simulink model "LEGO_SW_simp"  (R2023a)
settings: Solver=FixedStepAuto  StartTime=0.0  StopTime=45  FixedStep=1e-3  RelTol=1e-3  EnableMultiTasking=on
values from neighbouring files (symbols this model uses):
  A1 = [0,0,1,0 ... (first row only)    [run_LEGO_SW.m]
  A2 = [0,1;0,-W^2/(2*R^2)*(Kfrac+b+b_bar)/Denom]    [run_LEGO_SW.m]
  B1 = [0;0;2*(M*R*L+M*L^2+Jpsi)*Kt/Rdc/q;-2*((2*m+M)*R^2+2*J+M*R*L)*Kt/Rdc/q]    [run_LEGO_SW.m]
  B2 = [0;-W/R*Kt/Rdc/Denom]    [run_LEGO_SW.m]
  C1 = [1,0,0,0;0,0,0,1]    [run_LEGO_SW.m]
  C2 = [1,0]    [run_LEGO_SW.m]
  D1 = [0;0]    [run_LEGO_SW.m]
  D2 = 0    [run_LEGO_SW.m]
  KPphi = 6    [run_LEGO_SW.m]
undefined symbols (not defined in the file or in its folder): Kpp, sigbuilder_block
settings Model: Creator=KostasM  LastModifiedBy=lab5
settings SolverCC: AlgebraicLoopSolver=TrustRegion
settings DataIOCC: LimitDataPoints=on  ReturnWorkspaceOutputs=off
settings OptimizationCC: LifeSpan=inf
settings DebuggingCC: UnconnectedInputMsg=warning  UnconnectedOutputMsg=warning  UnconnectedLineMsg=warning  AllowSymbolicDim=off  SFUnexpectedBacktrackingDiag=warning  SFNoUnconditionalDefaultTransitionDiag=warning  SFExecutionAtInitializationDiag=none  ArithmeticOperatorsInVariantConditions=warning
settings ModelReferenceCC: EnableRefExpFcnMdlSchedulingChecks=on  PropagateSignalLabelsOutOfModel=off
settings SFSimCC: SimUseLocalCustomCode=off  CustomCodeUndefinedFunction=UseInterfaceOnly
settings RTWCC: RTWUseLocalCustomCode=off  DLArmComputeVersion=19.05
settings CodeAppCC: StateflowObjectComments=on
settings GRTTargetCC: TargetLangStandard=C89/C90 (ANSI)
settings ConfigComp: CovMetricSettings=dw  CovSaveCumulativeToWorkspaceVar=on  CovSaveSingleToWorkspaceVar=on  CovExternalEMLEnable=off

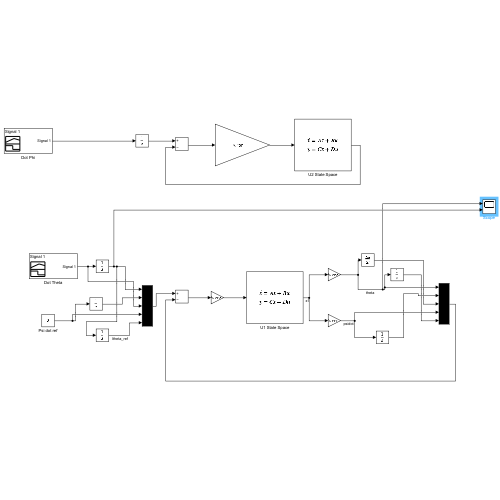
[thumbnail: Simulink's stored preview of the top-level diagram]
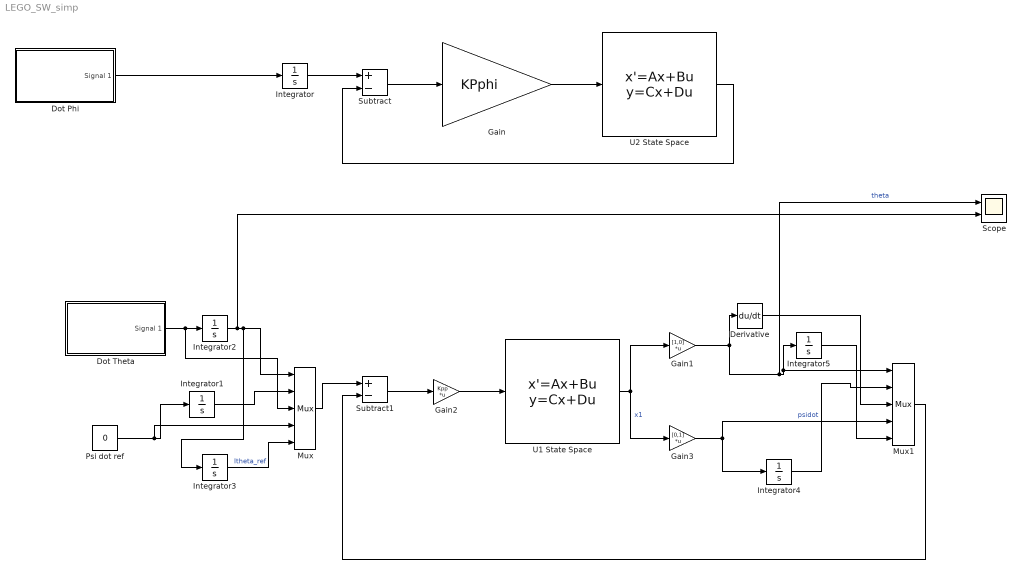
== system LEGO_SW_simp ==
  Derivative : Derivative
  Dot Phi : Subsystem  Tag=STV Subsys  LoadFcn=sigbuilder_block('load');  StartFcn=sigbuilder_block('start');  StopFcn=sigbuilder_block('stop');  ClipboardFcn=sigbuilder_block('clipboard');  mask(Sigbuilder block){tuvar=[0:10]}
      mask help: Sigbuilder GUI
      mask init:
      | if ~strcmp(get_param(bdroot(gcbh),'SimulationStatus'),'stopped') tuvar = sigbuilder_block('maskInit'); end
      settings: CopyFcn=sigbuilder_block('copy');  DeleteFcn=sigbuilder_block('delete');  ModelCloseFcn=sigbuilder_block('modelClose');  PreSaveFcn=sigbuilder_block('preSave');  PauseFcn=sigbuilder_block('pause')  ContinueFcn=sigbuilder_block('continue')  NameChangeFcn=sigbuilder_block('namechange');  OpenFcn=sigbuilder_block('open',[181.5 38.5 516 349.5 ]);  CloseFcn=sigbuilder_block('close');
      mask Display: plot(0, 0, 100, 100,[2, 2, 32, 32, 2], [68, 8, 8, 68, 68],[32, 2], [38, 38], [32, 19, 2],[53, 60, 44], [32, 17, 17, 2],[16, 16, 31, 31]);txt = getActiveGroup(gcbh);text(2, 100, txt,'verticalAlignment', 'top');
  Dot Theta : Subsystem  Tag=STV Subsys  LoadFcn=sigbuilder_block('load',[181.5 38.5 516 349.5 ]);  StartFcn=sigbuilder_block('start');  StopFcn=sigbuilder_block('stop');  ClipboardFcn=sigbuilder_block('clipboard');  mask(Sigbuilder block){tuvar=[0:10]}
      mask help: Sigbuilder GUI
      mask init:
      | if ~strcmp(get_param(bdroot(gcbh),'SimulationStatus'),'stopped') tuvar = sigbuilder_block('maskInit'); end
      settings: CopyFcn=sigbuilder_block('copy');  DeleteFcn=sigbuilder_block('delete');  ModelCloseFcn=sigbuilder_block('modelClose');  PreSaveFcn=sigbuilder_block('preSave');  PauseFcn=sigbuilder_block('pause')  ContinueFcn=sigbuilder_block('continue')  NameChangeFcn=sigbuilder_block('namechange');  OpenFcn=sigbuilder_block('open',[181.5 38.5 516 349.5 ]);  CloseFcn=sigbuilder_block('close');
      mask Display: plot(0, 0, 100, 100,[2, 2, 32, 32, 2], [68, 8, 8, 68, 68],[32, 2], [38, 38], [32, 19, 2],[53, 60, 44], [32, 17, 17, 2],[16, 16, 31, 31]);txt = getActiveGroup(gcbh);text(2, 100, txt,'verticalAlignment', 'top');
  Gain : Gain  Gain=KPphi
  Gain1 : Gain  Gain=[1,0]  Multiplication=Matrix(K*u) (u vector)
  Gain2 : Gain  Gain=Kpp  Multiplication=Matrix(K*u) (u vector)
  Gain3 : Gain  Gain=[0,1]  Multiplication=Matrix(K*u) (u vector)
  Integrator{,1..5} (6 alike) : Integrator
  Mux : Mux  Inputs=5
  Mux1 : Mux  Inputs=5
  Psi dot ref : Constant  Value=0
  Scope : Scope  NumInputPorts=2
  Subtract : Sum  Inputs=+-
  Subtract1 : Sum  Inputs=+-
  U1 State Space : StateSpace  A=A1  B=B1  C=C1  D=D1  InitialCondition=0
  U2 State Space : StateSpace  A=A2  B=B2  C=C2  D=D2  InitialCondition=0
  wires:
  Dot Phi/1(Signal 1) -> Integrator/1
  Dot Theta/1(Signal 1) -> Mux/3, Integrator2/1
  Integrator/1 -> Subtract/1
  Subtract/1 -> Gain/1
  Gain/1 -> U2 State Space/1
  U2 State Space/1 -> Subtract/2
  Psi dot ref/1 -> Mux/4, Integrator1/1
  Integrator2/1 -> Scope/2, Integrator3/1, Mux/1
  Mux/1 -> Subtract1/1
  Subtract1/1 -> Gain2/1
  Integrator1/1 -> Mux/2
  Integrator3/1 -> Mux/5  "Itheta_ref"
  Gain1/1 -> Derivative/1, Scope/1, Mux1/1, Integrator5/1  "theta"
  Gain3/1 -> Mux1/4, Integrator4/1  "psidot"
  Integrator4/1 -> Mux1/2
  Derivative/1 -> Mux1/3
  Integrator5/1 -> Mux1/5
  Mux1/1 -> Subtract1/2
  Gain2/1 -> U1 State Space/1
  U1 State Space/1 -> Gain1/1, Gain3/1  "x1"

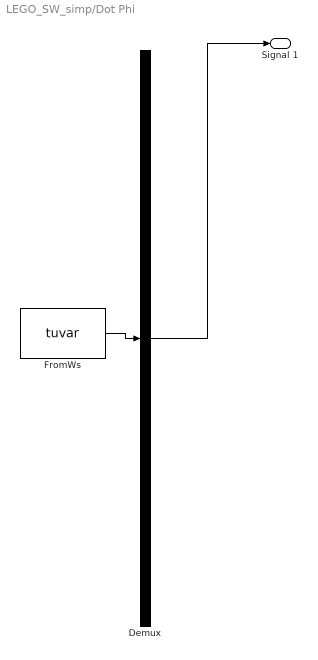
== system LEGO_SW_simp/Dot Phi ==
  Demux : Demux  Tag=STV Demux  Outputs=1
      settings: DisplayOption=none
  FromWs : FromWorkspace  Tag=STV FromWs  VariableName=tuvar
      SigBuilderData=|
      | common.afterFinalStr = 'Extrapolate'
      | common.sampleTime = 0
      | dataSet.timeRange = [0 25]
      | dataSet.name = 'Signal 1'
      | sbobj.Groups.Name = 'Signal 1'
      | sbobj.Groups.Signals.Name = 'Signal 1'
      | sbobj.Groups.Signals.XData = [0 12.5 12.5 25]
      | sbobj.Groups.Signals.YData = [0 0 1 1]
      | sbobj.Groups.TimeRange = [0 25]
  Signal 1 : Outport  Tag=STV Outport
  wires:
  FromWs/1 -> Demux/1
  Demux/1 -> Signal 1/1

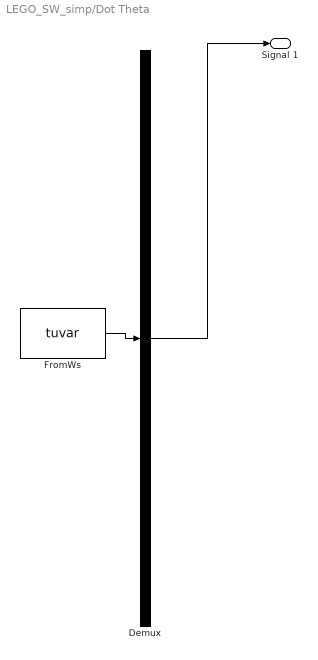
== system LEGO_SW_simp/Dot Theta ==
  Demux : Demux  Tag=STV Demux  Outputs=1
      settings: DisplayOption=none
  FromWs : FromWorkspace  Tag=STV FromWs  VariableName=tuvar
      SigBuilderData=|
      | common.afterFinalStr = 'Extrapolate'
      | common.sampleTime = 0
      | dataSet.timeRange = [0 25]
      | dataSet.name = 'Signal 1'
      | sbobj.Groups.Name = 'Signal 1'
      | sbobj.Groups.Signals.Name = 'Signal 1'
      | sbobj.Groups.Signals.XData = [0 12.5 12.5 25]
      | sbobj.Groups.Signals.YData = [0 0 1 1]
      | sbobj.Groups.TimeRange = [0 25]
  Signal 1 : Outport  Tag=STV Outport
  wires:
  FromWs/1 -> Demux/1
  Demux/1 -> Signal 1/1
